simulink library "calcDesTanRoll_cl"  (R2020a)
settings: Solver=VariableStepAuto  StartTime=0.0  StopTime=10.0  RelTol=1e-3
libraries: calcDesTanRollAng_ul x1, calcTurnAngleInTangentFrame_ul x1, findClosestPathParameter_ul x1, setTargetPathLoc_ul x1
settings Model: Creator=Ayaz  LastModifiedBy=Ayaz

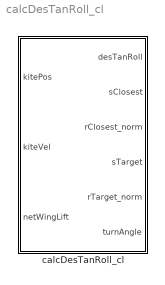
== system calcDesTanRoll_cl ==
  calcDesTanRoll_cl : Subsystem  mask{fltC=0}
      mask prompts: fltC "Path following controller object"

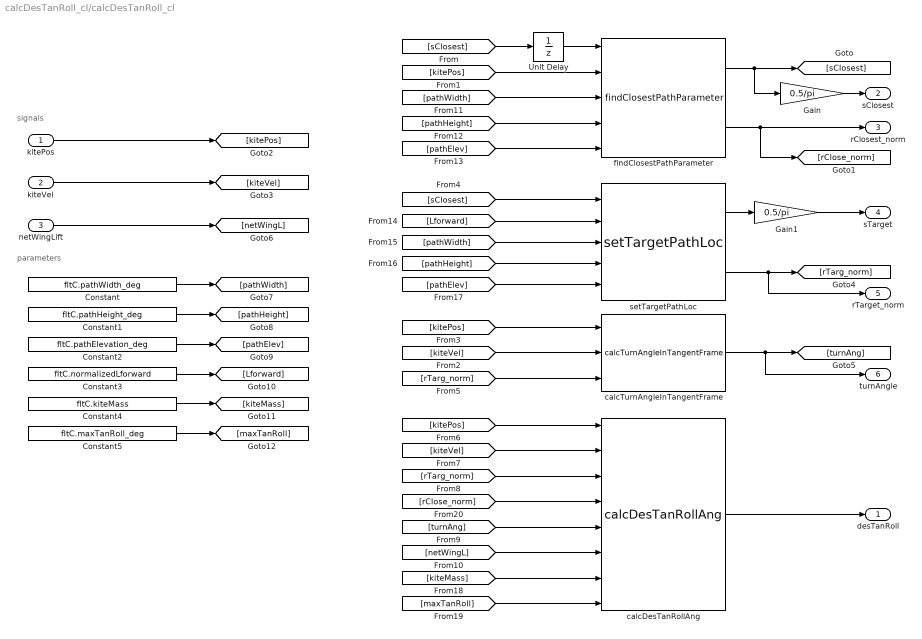
== system calcDesTanRoll_cl/calcDesTanRoll_cl ==
  note: parameters
  note: signals
  kitePos : Inport
  kiteVel : Inport  Port=2
  netWingLift : Inport  Port=3
  Constant : Constant  Value=fltC.pathWidth_deg
  Constant1 : Constant  Value=fltC.pathHeight_deg
  Constant2 : Constant  Value=fltC.pathElevation_deg
  Constant3 : Constant  Value=fltC.normalizedLforward
  Constant4 : Constant  Value=fltC.kiteMass
  Constant5 : Constant  Value=fltC.maxTanRoll_deg
  Gain : Gain  Gain=0.5/pi
  Gain1 : Gain  Gain=0.5/pi
  Unit Delay : UnitDelay  InitialCondition=fltC.initPathParameter  SampleTime=-1  HasFrameUpgradeWarning=on
  calcDesTanRollAng : calcDesTanRollAng_ul/calcDesTanRollAng  SystemSampleTime=-1  Latency=0  AutoFrameSizeCalculation=off
  calcTurnAngleInTangentFrame : calcTurnAngleInTangentFrame_ul/calcTurnAngleInTangentFrame  SystemSampleTime=-1  Latency=0  AutoFrameSizeCalculation=off
  findClosestPathParameter : findClosestPathParameter_ul/findClosestPathParameter  SystemSampleTime=-1  Latency=0  AutoFrameSizeCalculation=off
  setTargetPathLoc : setTargetPathLoc_ul/setTargetPathLoc  SystemSampleTime=-1  Latency=0  AutoFrameSizeCalculation=off
  desTanRoll : Outport
  sClosest : Outport  Port=2
  rClosest_norm : Outport  Port=3
  sTarget : Outport  Port=4
  rTarget_norm : Outport  Port=5
  turnAngle : Outport  Port=6
  wires:
  calcDesTanRollAng/1 -> desTanRoll/1
  Unit Delay/1 -> findClosestPathParameter/1
  findClosestPathParameter/1 -> [sClosest], Gain/1
  [sClosest] -> Unit Delay/1
  kitePos/1 -> [kitePos]
  [kitePos] -> findClosestPathParameter/2
  kiteVel/1 -> [kiteVel]
  [kiteVel] -> calcTurnAngleInTangentFrame/2
  [kitePos] -> calcTurnAngleInTangentFrame/1
  [sClosest] -> setTargetPathLoc/1
  setTargetPathLoc/2 -> rTarget_norm/1, [rTarg_norm]
  [rTarg_norm] -> calcTurnAngleInTangentFrame/3
  [kitePos] -> calcDesTanRollAng/1
  [kiteVel] -> calcDesTanRollAng/2
  [rTarg_norm] -> calcDesTanRollAng/3
  calcTurnAngleInTangentFrame/1 -> turnAngle/1, [turnAng]
  netWingLift/1 -> [netWingL]
  Constant/1 -> [pathWidth]
  Constant1/1 -> [pathHeight]
  Constant2/1 -> [pathElev]
  [pathWidth] -> findClosestPathParameter/3
  [pathHeight] -> findClosestPathParameter/4
  [pathElev] -> findClosestPathParameter/5
  Constant3/1 -> [Lforward]
  [Lforward] -> setTargetPathLoc/2
  [pathWidth] -> setTargetPathLoc/3
  [pathHeight] -> setTargetPathLoc/4
  [pathElev] -> setTargetPathLoc/5
  Constant4/1 -> [kiteMass]
  Constant5/1 -> [maxTanRoll]
  Gain/1 -> sClosest/1
  findClosestPathParameter/2 -> [rClose_norm], rClosest_norm/1
  setTargetPathLoc/1 -> Gain1/1
  Gain1/1 -> sTarget/1
  [maxTanRoll] -> calcDesTanRollAng/8
  [kiteMass] -> calcDesTanRollAng/7
  [netWingL] -> calcDesTanRollAng/6
  [turnAng] -> calcDesTanRollAng/5
  [rClose_norm] -> calcDesTanRollAng/4
